simulink model "position_estimator_G"  (R2021a)
settings: Solver=VariableStepDiscrete  StartTime=0.0  StopTime=10.0  RelTol=1e-3
values from neighbouring files (symbols this model uses):
  a33 = 1/(Ts*wa + 1)    (= 0.997388842117)    [dev_position_estimator.m]    (also in eval_logs.m = 0.998744940093; position_estimator.m = G(3,3); position_estimator_debug_bf.m = 1 / (Ts*wa + 1))
  G = G0 * tf(num, den)    [check_pade.m]    (also in dev_position_estimator.m = [[1, a12,   0, Ts*a12, k1]; eval_besself.m = tf(b, a); eval_filter_poles.m = get_filter('pt3', f0, Ts); eval_logs.m = [[1, a12,   0, Ts*a12, k1])
  nd_pos = 9    [dev_position_estimator.m]    (also in eval_logs.m = 3; test_position_estimator.m)
  Ts = 1/40    (= 0.025)    [check_median.m]    (also in check_pade.m; check_pt3_init.m; dev_position_estimator.m = 0.00833333333333; eval_filter_poles.m = 0.01)
settings Model: Creator=pmic  LastModifiedBy=pmic

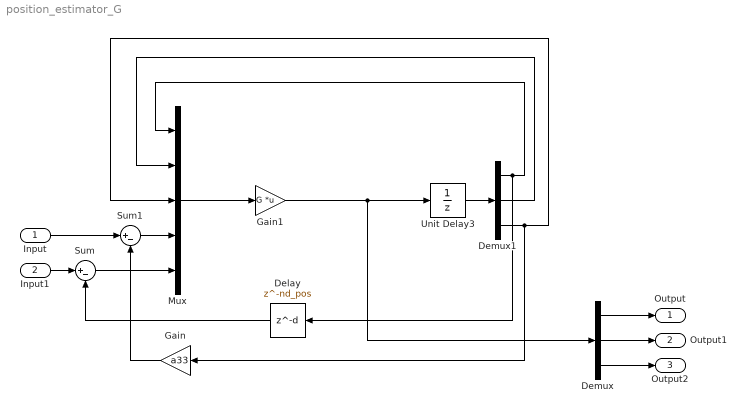
== system position_estimator_G ==
  Input : Inport
  Input1 : Inport  Port=2
  Delay : Delay  DelayLength=nd_pos  SampleTime=Ts
  Demux : Demux  Outputs=3
  Demux1 : Demux  Outputs=3
  Gain : Gain  Gain=a33
  Gain1 : Gain  Gain=G  Multiplication=Matrix(K*u)
  Mux : Mux  Inputs=5
  Sum : Sum  Inputs=|+-
  Sum1 : Sum  Inputs=|+-
  Unit Delay3 : UnitDelay  SampleTime=Ts  HasFrameUpgradeWarning=on
  Output : Outport
  Output1 : Outport  Port=2
  Output2 : Outport  Port=3
  wires:
  Demux/1 -> Output/1
  Demux/2 -> Output1/1
  Demux/3 -> Output2/1
  Unit Delay3/1 -> Demux1/1
  Input1/1 -> Sum/1
  Gain/1 -> Sum1/2
  Sum/1 -> Mux/5
  Input/1 -> Sum1/1
  Demux1/1 -> Mux/1, Delay/1
  Demux1/2 -> Mux/2
  Sum1/1 -> Mux/4
  Mux/1 -> Gain1/1
  Gain1/1 -> Demux/1, Unit Delay3/1
  Demux1/3 -> Gain/1, Mux/3
  Delay/1 -> Sum/2
